simulink model "variant_drag"  (Simulink 7.9)
settings: Solver=ode45  StartTime=0.0  StopTime=10.0  RelTol=1e-3
libraries: aerolibatmos2 x1
settings Model: Creator=wcampbel  LastModifiedBy=wcampbel

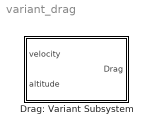
== system variant_drag ==
  Drag: Variant Subsystem : Subsystem  Variant=on  OverrideUsingVariant=A == 2

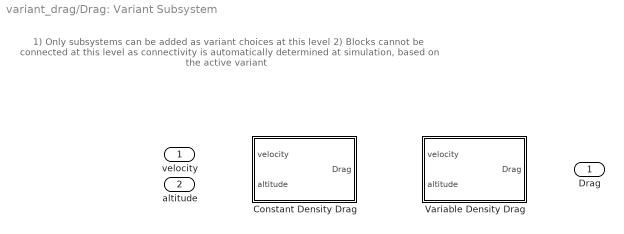
== system variant_drag/Drag: Variant Subsystem ==
  note: 1) Only subsystems can be added as variant choices at this level
      | 2) Blocks cannot be connected at this level as connectivity is
      | automatically determined at simulation, based on the active variant
  velocity : Inport
  altitude : Inport  Port=2
  Constant Density Drag : Subsystem  VariantObject=A == 1  mask(Constant Density Drag Model){rho=1.2, Cd=0.333, A=1.5}
      mask prompts: rho "Air Density [kg/m^3]"; Cd "Drag Coefficient [N/A]"; A "Reference Area [m^2]"
      mask help: Applies the equation D = -0.5*rho*Cd*A*V^2. V is designed to be a velocity vector of length 3.
  Variable Density Drag : Subsystem  VariantObject=A == 2  mask(Variable Density Drag Model){Cd=0.333, A=1.5}
      mask prompts: Cd "Drag Coefficient [N/A]"; A "Reference Area [m^2]"
      mask help: Applies the equation D = -0.5*rho*Cd*A*V^2 where rho is a function of altitude. V is designed to be a velocity vector of length 3.
  Drag : Outport

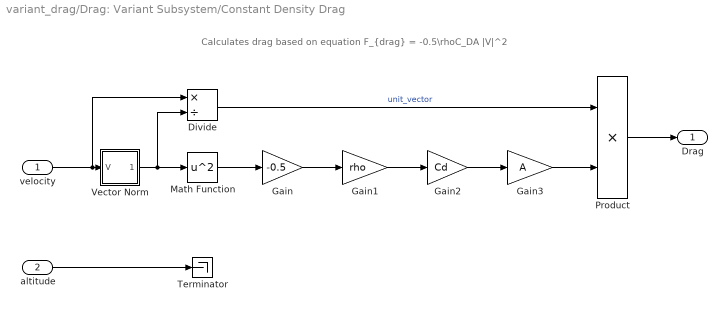
== system variant_drag/Drag: Variant Subsystem/Constant Density Drag ==
  note: Calculates drag based on equation F_{drag} = -0.5\rhoC_DA |V|^2
  velocity : Inport
  altitude : Inport  Port=2
  Divide : Product  Inputs=*/
  Gain : Gain  Gain=-0.5
  Gain1 : Gain  Gain=rho
  Gain2 : Gain  Gain=Cd
  Gain3 : Gain  Gain=A
  Math Function : Math  Operator=square  SaturateOnIntegerOverflow=on
  Product : Product  RndMeth=Zero
  Terminator : Terminator
  Vector Norm : Subsystem
      mask Type: Vector Norm
      mask Description: Calculates the magnitude of a vector of arbitrary length.
      mask Help:
      | Will Campbell
      | Senior Application Engineer
      | The MathWorks, Inc.
      | 14 Nov 2007
      mask Display: disp('|\bfV|','texmode','on')
  Drag : Outport
  wires:
  altitude/1 -> Terminator/1
  velocity/1 -> Vector Norm/1(V), Divide/1
  Vector Norm/1(norm) -> Math Function/1, Divide/2
  Gain/1 -> Gain1/1
  Gain1/1 -> Gain2/1
  Gain2/1 -> Gain3/1
  Math Function/1 -> Gain/1
  Divide/1 -> Product/1  "unit_vector"
  Gain3/1 -> Product/2
  Product/1 -> Drag/1

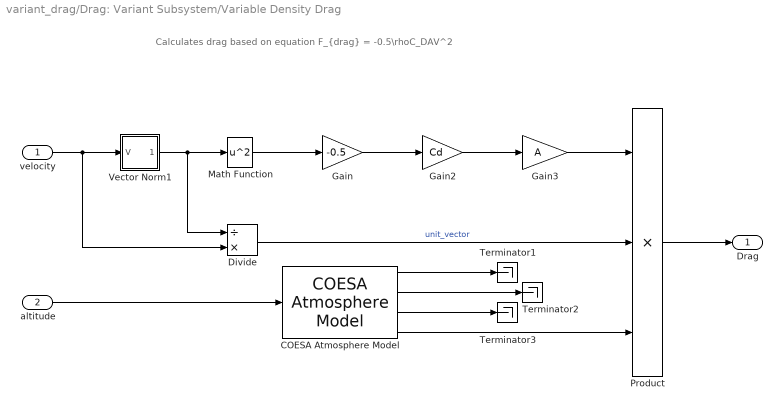
== system variant_drag/Drag: Variant Subsystem/Variable Density Drag ==
  note: Calculates drag based on equation F_{drag} = -0.5\rhoC_DAV^2
  velocity : Inport
  altitude : Inport  Port=2
  COESA Atmosphere Model : aerolibatmos2/COESA Atmosphere Model  units=Metric (MKS)  spec=1976 COESA-extended U.S. Standard Atmosphere  model=Profile  profile_var=High temperature  profile_percent=1%  profile_alt=5 km (16404 ft)  envelope_var=High temperature  envelope_percent=1%  action=None
  Divide : Product  Inputs=/*
  Gain : Gain  Gain=-0.5
  Gain2 : Gain  Gain=Cd
  Gain3 : Gain  Gain=A
  Math Function : Math  Operator=square  SaturateOnIntegerOverflow=on
  Product : Product  Inputs=3  RndMeth=Zero
  Terminator1 : Terminator
  Terminator2 : Terminator
  Terminator3 : Terminator
  Vector Norm1 : Subsystem
      mask Type: Vector Norm
      mask Description: Calculates the magnitude of a vector of arbitrary length.
      mask Help:
      | Will Campbell
      | Senior Application Engineer
      | The MathWorks, Inc.
      | 14 Nov 2007
      mask Display: disp('|\bfV|','texmode','on')
  Drag : Outport
  wires:
  altitude/1 -> COESA Atmosphere Model/1
  velocity/1 -> Divide/2, Vector Norm1/1(V)
  Math Function/1 -> Gain/1
  Gain2/1 -> Gain3/1
  COESA Atmosphere Model/1 -> Terminator1/1
  COESA Atmosphere Model/2 -> Terminator2/1
  COESA Atmosphere Model/3 -> Terminator3/1
  Gain/1 -> Gain2/1
  Vector Norm1/1(norm) -> Math Function/1, Divide/1
  Product/1 -> Drag/1
  Gain3/1 -> Product/1
  Divide/1 -> Product/2  "unit_vector"
  COESA Atmosphere Model/4 -> Product/3

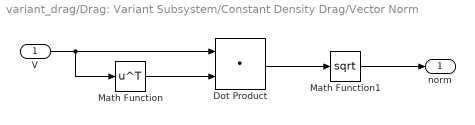
== system variant_drag/Drag: Variant Subsystem/Constant Density Drag/Vector Norm ==
  V : Inport
  Dot Product : DotProduct  InputSameDT=on  OutDataTypeStr=Inherit: Inherit via internal rule
  Math Function : Math  Operator=transpose  SaturateOnIntegerOverflow=on
  Math Function1 : Math  Operator=sqrt  SaturateOnIntegerOverflow=on
  norm : Outport
  wires:
  V/1 -> Dot Product/1, Math Function/1
  Math Function/1 -> Dot Product/2
  Dot Product/1 -> Math Function1/1
  Math Function1/1 -> norm/1

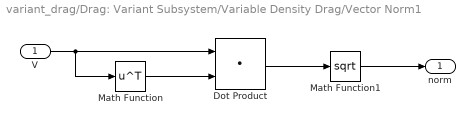
== system variant_drag/Drag: Variant Subsystem/Variable Density Drag/Vector Norm1 ==
  V : Inport
  Dot Product : DotProduct  InputSameDT=on  OutDataTypeStr=Inherit: Inherit via internal rule
  Math Function : Math  Operator=transpose  SaturateOnIntegerOverflow=on
  Math Function1 : Math  Operator=sqrt  SaturateOnIntegerOverflow=on
  norm : Outport
  wires:
  Math Function1/1 -> norm/1
  Dot Product/1 -> Math Function1/1
  Math Function/1 -> Dot Product/2
  V/1 -> Math Function/1, Dot Product/1
